simulink model "modele_simulink_Matlab_fnc"  (Simulink 7.0)
settings: Solver=ode3  StartTime=0.0  StopTime=10.0  FixedStep=1e-3  RelTol=1e-3
values from neighbouring files (symbols this model uses):
  pneu = [1.712 -66.87 1169 851.9 4.943 0.01399 -0.1911 1 0.972 0 0.186 0.22 ... (35 elements, 1x35)]    [Correcteur.mat]    (also in DVinitialisation.m = [a0,a1,a2,a3,a4,a5,a6,a7,am0,am1,am2,am3,am4,am5,am6,am7,am8; pacejka_BE_Matlab_fnc.m = in(5:end); param_pneu_P1_OK.m = [a0,a1,a2,a3,a4,a5,a6,a7,am0,am1,am2,am3,am4,am5,am6,am7,am8)
settings Model: Creator=Rizzo  LastModifiedBy=MOREAU

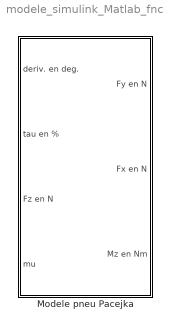
== system modele_simulink_Matlab_fnc ==
  Modele pneu Pacejka : Subsystem

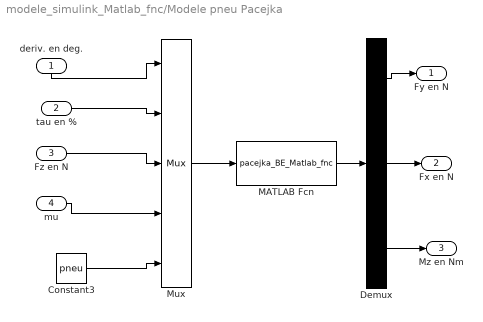
== system modele_simulink_Matlab_fnc/Modele pneu Pacejka ==
  deriv. en deg. : Inport  Orientation=down
  tau en % : Inport  Port=2
  Fz en N : Inport  Port=3
  mu : Inport  Port=4
  Constant3 : Constant  Value=pneu  OutDataType=sfix(16)  OutScaling=2^0
  Demux : Demux  Outputs=3
  MATLAB Fcn : MATLABFcn  MATLABFcn=pacejka_BE_Matlab_fnc  OutputDimensions=3
  Mux : Mux  Inputs=5
  Fy en N : Outport
  Fx en N : Outport  Port=2
  Mz en Nm : Outport  Port=3
  wires:
  MATLAB Fcn/1 -> Demux/1
  Mux/1 -> MATLAB Fcn/1
  deriv. en deg./1 -> Mux/1
  Demux/1 -> Fy en N/1
  Demux/2 -> Fx en N/1
  Demux/3 -> Mz en Nm/1
  tau en %/1 -> Mux/2
  Fz en N/1 -> Mux/3
  mu/1 -> Mux/4
  Constant3/1 -> Mux/5
